simulink model "iiwa_IK_FABRIK_ROS (bkp)"  (R2016b)
settings: Solver=FixedStepAuto  StartTime=0.0  StopTime=inf  FixedStep=0.05  RelTol=1e-3
model workspace (MAT data in the model file):
  SL_ROS_VariableLengthArrays_MaxSizes.CommonInfo.ArrayTruncateAction = 'EmitWarning'
  SL_ROS_VariableLengthArrays_MaxSizes.MsgTypeMap = containers.Map
  SL_ROS_VariableLengthArrays_MaxSizes.MsgTypeMap.serialization.keys = {'nav_msgs/Path', 'sensor_msgs/JointState'}
  SL_ROS_VariableLengthArrays_MaxSizes.MsgTypeMap.serialization.values{1}.PropertyName = 'Poses'
  SL_ROS_VariableLengthArrays_MaxSizes.MsgTypeMap.serialization.values{1}.DataType = 'geometry_msgs/PoseStamped'
  SL_ROS_VariableLengthArrays_MaxSizes.MsgTypeMap.serialization.values{1}.MaxLength = 330
  SL_ROS_VariableLengthArrays_MaxSizes.MsgTypeMap.serialization.values{2}(1).PropertyName = 'Name'
  SL_ROS_VariableLengthArrays_MaxSizes.MsgTypeMap.serialization.values{2}(1).DataType = 'std_msgs/String'
  SL_ROS_VariableLengthArrays_MaxSizes.MsgTypeMap.serialization.values{2}(1).MaxLength = 30
  SL_ROS_VariableLengthArrays_MaxSizes.MsgTypeMap.serialization.values{2}(2).PropertyName = 'Position'
  SL_ROS_VariableLengthArrays_MaxSizes.MsgTypeMap.serialization.values{2}(2).DataType = 'double'
  SL_ROS_VariableLengthArrays_MaxSizes.MsgTypeMap.serialization.values{2}(2).MaxLength = 128
  SL_ROS_VariableLengthArrays_MaxSizes.MsgTypeMap.serialization.values{2}(3).PropertyName = 'Velocity'
  SL_ROS_VariableLengthArrays_MaxSizes.MsgTypeMap.serialization.values{2}(3).DataType = 'double'
  SL_ROS_VariableLengthArrays_MaxSizes.MsgTypeMap.serialization.values{2}(3).MaxLength = 128
  SL_ROS_VariableLengthArrays_MaxSizes.MsgTypeMap.serialization.values{2}(4).PropertyName = 'Effort'
  SL_ROS_VariableLengthArrays_MaxSizes.MsgTypeMap.serialization.values{2}(4).DataType = 'double'
  SL_ROS_VariableLengthArrays_MaxSizes.MsgTypeMap.serialization.values{2}(4).MaxLength = 128
  SL_ROS_VariableLengthArrays_MaxSizes.MsgTypeMap.serialization.uniformity = 0
  SL_ROS_VariableLengthArrays_MaxSizes.MsgTypeMap.serialization.keyType = 'char'
  SL_ROS_VariableLengthArrays_MaxSizes.MsgTypeMap.serialization.valueType = 'any'
libraries: robotlib x7
(part 1 of 2)
settings Model: Creator=ram  LastModifiedBy=ram

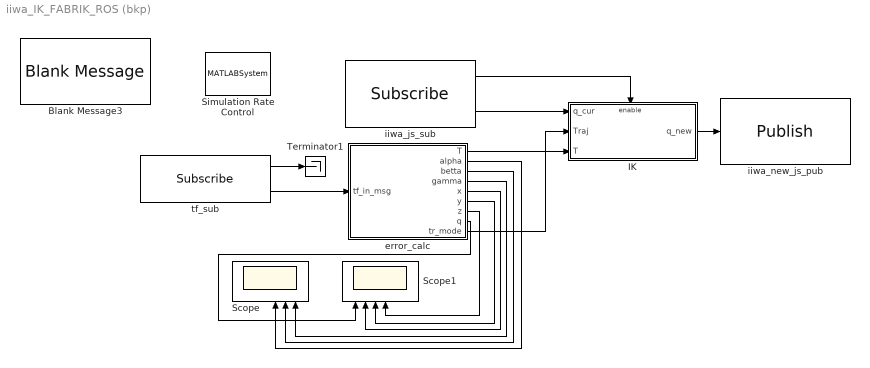
== system iiwa_IK_FABRIK_ROS (bkp) ==
  Blank Message3 : robotlib/Blank Message  SourceLibraryInfo=This block requires Robotics System Toolbox  messageType=tf2_msgs/TFMessage  SampleTime=inf
  IK : Subsystem
  Scope : Scope  NumInputPorts=6
  Scope1 : Scope  NumInputPorts=6
  Simulation Rate Control : MATLABSystem  System=ExampleHelperSimulationRateControl  SampleTime=0.05
      mask Type: ExampleHelperSimulationRateControl
      mask Display: disp('Rate Control');
  Terminator1 : Terminator
  error_calc : MATLAB Function  TreatAsAtomicUnit=on
  iiwa_js_sub : robotlib/Subscribe  SourceLibraryInfo=This block requires Robotics System Toolbox  topicSource=Select from ROS network  topic=/joint_states  messageType=sensor_msgs/JointState  sampleTime=-1  messageQueueLength=1
  iiwa_new_js_pub : robotlib/Publish  SourceLibraryInfo=This block requires Robotics System Toolbox  topicSource=Select from ROS network  topic=/arm_state  messageType=sensor_msgs/JointState  messageQueueLength=5
  tf_sub : robotlib/Subscribe  SourceLibraryInfo=This block requires Robotics System Toolbox  topicSource=Select from ROS network  topic=/tf  messageType=tf2_msgs/TFMessage  sampleTime=-1  messageQueueLength=1
  wires:
  tf_sub/2 -> error_calc/1(tf_in_msg)
  tf_sub/1 -> Terminator1/1
  iiwa_js_sub/1 -> IK/Enable
  error_calc/1(T) -> IK/3(T)
  iiwa_js_sub/2 -> IK/1(q_cur)
  IK/1(q_new) -> iiwa_new_js_pub/1
  error_calc/5(x) -> Scope1/2
  error_calc/6(y) -> Scope1/3
  error_calc/7(z) -> Scope1/4
  error_calc/2(alpha) -> Scope/4
  error_calc/3(betta) -> Scope/5
  error_calc/4(gamma) -> Scope/6
  error_calc/8(q) -> Scope1/1
  error_calc/9(tr_mode) -> IK/2(Traj)

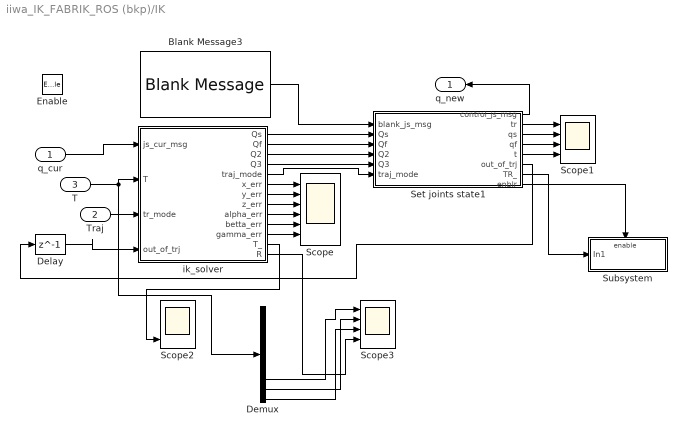
== system iiwa_IK_FABRIK_ROS (bkp)/IK ==
  q_cur : Inport
  Traj : Inport  Port=2
  T : Inport  Port=3
  Enable : EnablePort
  Blank Message3 : robotlib/Blank Message  SourceLibraryInfo=This block requires Robotics System Toolbox  messageType=sensor_msgs/JointState  SampleTime=inf
  Delay : Delay  DelayLength=1
  Demux : Demux  Outputs=10
  Scope : Scope  NumInputPorts=6
  Scope1 : Scope  NumInputPorts=4
  Scope2 : Scope  NumInputPorts=4
  Scope3 : Scope  NumInputPorts=4
  Set joints state1 : MATLAB Function  TreatAsAtomicUnit=on
  Subsystem : Subsystem
  ik_solver : MATLAB Function  TreatAsAtomicUnit=on
  q_new : Outport
  wires:
  T/1 -> Demux/1, ik_solver/2(T)
  q_cur/1 -> ik_solver/1(js_cur_msg)
  Blank Message3/1 -> Set joints state1/1(blank_js_msg)
  Set joints state1/1(control_js_msg) -> q_new/1
  ik_solver/2(Qf) -> Set joints state1/3(Qf)
  ik_solver/6(x_err) -> Scope/1
  ik_solver/7(y_err) -> Scope/2
  ik_solver/8(z_err) -> Scope/3
  ik_solver/9(alpha_err) -> Scope/4
  ik_solver/10(betta_err) -> Scope/5
  ik_solver/11(gamma_err) -> Scope/6
  Traj/1 -> ik_solver/3(tr_mode)
  ik_solver/5(traj_mode) -> Set joints state1/6(traj_mode)
  Set joints state1/6(out_of_trj) -> Delay/1
  ik_solver/1(Qs) -> Set joints state1/2(Qs)
  ik_solver/3(Q2) -> Set joints state1/4(Q2)
  ik_solver/4(Q3) -> Set joints state1/5(Q3)
  Delay/1 -> ik_solver/4(out_of_trj)
  Set joints state1/2(tr) -> Scope1/1
  Set joints state1/3(qs) -> Scope1/2
  Set joints state1/4(qf) -> Scope1/3
  Set joints state1/5(t) -> Scope1/4
  Set joints state1/7(TR_) -> Subsystem/1(In1)
  Set joints state1/8(enblr) -> Subsystem/Enable
  ik_solver/12(T_) -> Scope2/4
  ik_solver/13(R) -> Scope3/4
  Demux/10 -> Scope3/3
  Demux/8 -> Scope3/1
  Demux/9 -> Scope3/2

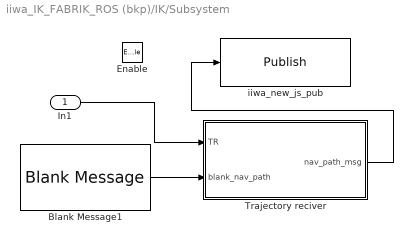
== system iiwa_IK_FABRIK_ROS (bkp)/IK/Subsystem ==
  In1 : Inport
  Enable : EnablePort
  Blank Message1 : robotlib/Blank Message  SourceLibraryInfo=This block requires Robotics System Toolbox  messageType=nav_msgs/Path  SampleTime=inf
  Trajectory reciver : MATLAB Function  TreatAsAtomicUnit=on
  iiwa_new_js_pub : robotlib/Publish  SourceLibraryInfo=This block requires Robotics System Toolbox  topicSource=Specify your own  topic=/tool_path  messageType=nav_msgs/Path  messageQueueLength=5
  wires:
  Blank Message1/1 -> Trajectory reciver/2(blank_nav_path)
  Trajectory reciver/1(nav_path_msg) -> iiwa_new_js_pub/1
  In1/1 -> Trajectory reciver/1(TR)

== matlab function iiwa_IK_FABRIK_ROS (bkp)/IK/Set joints state1 ==
  data: blank_js_msg input; Qs input; control_js_msg output Bus: SL_Bus_iiwa_IK_FABRIK_ROS_sensor_msgs_JointState; tr output; qs output; qf output; t output; Qf input double size=1 7; Q2 input; Q3 input; traj_mode input; out_of_trj output; TR_ output; enblr output
function [control_js_msg, tr, qs, qf, t, out_of_trj, TR_, enblr]   = fcn(blank_js_msg, Qs, Qf, Q2, Q3, traj_mode)

persistent on_traj;
if isempty(on_traj)
    on_traj = false;
end

persistent Qs_;
if isempty(Qs_)
    Qs_ = [0, 0, 0, 0, 0, 0];
end
qs = Qs_;
persistent Qf_;
if isempty(Qf_)
    Qf_ = [0, 0, 0, 0, 0, 0];
end
qf = Qf_;
persistent Q2_;
if isempty(Q2_)
    Q2_ = [0, 0, 0, 0, 0, 0];
end
persistent Q3_;
if isempty(Q3_)
    Q3_ = [0, 0, 0, 0, 0, 0];
end

persistent seq;
if isempty(seq)
    seq = 0;
end

persistent i;
if isempty(i)
    i = 0;
end

persistent TRth;
if isempty(TRth)
    TRth = zeros(300,6);
end

persistent TR;
if isempty(TR)
    TR = zeros(300,3);
end

enblr = 0;

out_of_trj = true;

str_array_of_jnames = {'iiwa_j1', 'iiwa_j2', 'iiwa_j3', 'iiwa_j4', 'iiwa_j5', 'iiwa_j6', 'iiwa_j7'};
control_js_msg = blank_js_msg;

th_num = length(str_array_of_jnames);
control_js_msg.Name_SL_Info.CurrentLength = uint32(th_num);

for idx=1:th_num
    str = str_array_of_jnames{idx};
    str_length = length(str);
    control_js_msg.Name(idx).Data(1:str_length) = uint8(str);
    control_js_msg.Name(idx).Data_SL_Info.CurrentLength = uint32(str_length);
end

if (traj_mode == false)
    control_js_msg.Position_SL_Info.CurrentLength = uint32(th_num);
    control_js_msg.Position(1) = double(Qf(1));
    control_js_msg.Position(2) = double(Qf(2));
    control_js_msg.Position(3) = double(Qf(3));
    control_js_msg.Position(4) = double(Qf(4));
    control_js_msg.Position(5) = double(Qf(5));
    control_js_msg.Position(6) = double(Qf(6));
    control_js_msg.Position(7) = double(Qf(7));

    control_js_msg.Header.Seq = uint32(seq);
    seq = seq + 1;
    tr = zeros(1,6);
    tr(1) = Qf(1); tr(2) = Qf(2); tr(3) = Qf(4); 
    tr(4) = Qf(5); tr(5) = Qf(6); tr(6) = Qf(7);
    t = 0;
    TR_ = zeros(300,3);
else
    if (on_traj == false)
        Qs_(1:2) = Qs(1:2); Qs_(3:6) = Qs(4:7);
        Q2_(1:2) = Q2(1:2); Q2_(3:6) = Q2(4:7);
        Q3_(1:2) = Q3(1:2); Q3_(3:6) = Q3(4:7);
        Qf_(1:2) = Qf(1:2); Qf_(3:6) = Qf(4:7);
        %%%%%%%%%%%%%%%%%%%%%%%%%%%%%%%%%%%%%%%%%%%%%%%%%%%%%
        enblr = 1;
        %TR_ = zeros(300,3);
        for j = 1:1:300
            tj = j/100;
            TRth(j,:) = traj434(2, Qs_', Q2_', Q3_', Qf_', tj);
            TR(j,:) = FK(TRth(j,1), TRth(j,2), 0.0, TRth(j,3), TRth(j,4), TRth(j,5), TRth(j,6));
            %plot3(TR(1:301,1), TR(1:301,2), TR(1:301,3));
        end
        %%%%%%%%%%%%%%%%%%%%%%%%%%%%%%%%%%%%%%%%%%%%%%%
        
        on_traj = true;
    end
    TR_ = TR;
    out_of_trj = false;
    
    t = i/100;
    tr = traj434(2, Qs_', Q2_', Q3_', Qf_', t);
    i = i + 1;
    if (i== 300)
        i = 0;
        out_of_trj = true;
        on_traj = false;
    end
    
    control_js_msg.Position_SL_Info.CurrentLength = uint32(th_num);
    control_js_msg.Position(1) = double(tr(1));
    control_js_msg.Position(2) = double(tr(2));
    control_js_msg.Position(3) = double(0.0);
    control_js_msg.Position(4) = double(tr(3));
    control_js_msg.Position(5) = double(tr(4));
    control_js_msg.Position(6) = double(tr(5));
    control_js_msg.Position(7) = double(tr(6));

    control_js_msg.Header.Seq = uint32(seq);
    seq = seq + 1;
    
end


end



function tr = traj434(in_t, in_qs, in_q2, in_q3, in_qf, t)%, in_dqs, in_dqf, in_ddqs, in_ddqf)
    
    n = 6;%numrows(in_qs);

    % Обнуление не заданных граничных условий
    %if nargin == 6 
        in_dqs  = zeros(1,n)'; in_dqf  = zeros(1,n)';
        in_ddqs = zeros(1,n)'; in_ddqf = zeros(1,n)';
    %end
    
    % интерполяция с интервалом в 10мс
    %itr_n = in_t*100;
    %t_step = 1/itr_n;
    
    % Соответствующая матрица из выражения 
    Am = [0  0  0  0  1  0  0   0   0   0   0   0   0   0;...
          0  0  0  1  0  0  0   0   0   0   0   0   0   0;...
          0  0  2  0  0  0  0   0   0   0   0   0   0   0;...
          1  1  1  1  1  0  0   0   0   0   0   0   0   0;...
          0  0  0  0  0  0  0   0   1   0   0   0   0   0;...
          4  3  2  1  0  0  0   -1  0   0   0   0   0   0;...
          12 6  2  0  0  0  -2  0   0   0   0   0   0   0;...
          0  0  0  0  0  1  1   1   1   0   0   0   0   0;...
          0  0  0  0  0  0  0   0   0   0   0   0   0   1;...
          0  0  0  0  0  3  2   1   0   0   0   0   -1  0;...
          0  0  0  0  0  6  2   0   0   0   0   -2  0   0;...
          0  0  0  0  0  0  0   0   0   1   1   1   1   1;...
          0  0  0  0  0  0  0   0   0   4   3   2   1   0;...
          0  0  0  0  0  0  0   0   0   12  6   2   0   0];
    Ami = inv(Am);
    
    % Определение полиномиальных коэффициентов для граничных условий
    % всех обобщенных координат A, скоростей dA и ускорений ddA
    A = ones(6,14);
    for i=1:n
        A(i,:)   = Ami*[in_qs(i); in_dqs(i); in_ddqs(i); in_q2(i); in_q2(i);0; 0; ...
                        in_q3(i); in_q3(i); 0; 0; in_qf(i); in_dqf(i); in_ddqf(i)];
    end
    
    % Вычисление значений интерполирующих полиномов по всей траектории
    tr = zeros(1,n);
    if t <= 1
        for i=1:n
            tr(1,i) = polyval(A(i,1:5),t);
        end
    end
    
    if (t > 1) && (t <= 2)
        for i=1:n
            tr(1,i) = polyval(A(i,6:9),(t-1));
        end
    end
    
    if (t > 2)
        for i=1:n
            tr(1,i) = polyval(A(i,10:14),(t-2));
        end
    end
end


function TRxyz = FK(th1, th2, th3, th4, th5, th6, th7)
d01 = 0.36;
d23 = 0.42;
d45 = 0.4;
d67 = 0.126;
H = [cos(th7)*(sin(th6)*(sin(th4)*(sin(th1)*sin(th3) - cos(th1)*cos(th2)*cos(th3)) - cos(th1)*cos(th4)*sin(th2)) - cos(th6)*(cos(th5)*(cos(th4)*(sin(th1)*sin(th3) - cos(th1)*cos(th2)*cos(th3)) + cos(th1)*sin(th2)*sin(th4)) + sin(th5)*(cos(th3)*sin(th1) + cos(th1)*cos(th2)*sin(th3)))) + sin(th7)*(sin(th5)*(cos(th4)*(sin(th1)*sin(th3) - cos(th1)*cos(th2)*cos(th3)) + cos(th1)*sin(th2)*sin(th4)) - cos(th5)*(cos(th3)*sin(th1) + cos(th1)*cos(th2)*sin(th3))), cos(th7)*(sin(th5)*(cos(th4)*(sin(th1)*sin(th3) - cos(th1)*cos(th2)*cos(th3)) + cos(th1)*sin(th2)*sin(th4)) - cos(th5)*(cos(th3)*sin(th1) + cos(th1)*cos(th2)*sin(th3))) - sin(th7)*(sin(th6)*(sin(th4)*(sin(th1)*sin(th3) - cos(th1)*cos(th2)*cos(th3)) - cos(th1)*cos(th4)*sin(th2)) - cos(th6)*(cos(th5)*(cos(th4)*(sin(th1)*sin(th3) - cos(th1)*cos(th2)*cos(th3)) + cos(th1)*sin(th2)*sin(th4)) + sin(th5)*(cos(th3)*sin(th1) + cos(th1)*cos(th2)*sin(th3)))),   cos(th6)*(sin(th4)*(sin(th1)*sin(th3) - cos(th1)*cos(th2)*cos(th3)) - cos(th1)*cos(th4)*sin(th2)) + sin(th6)*(cos(th5)*(cos(th4)*(sin(th1)*sin(th3) - cos(th1)*cos(th2)*cos(th3)) + cos(th1)*sin(th2)*sin(th4)) + sin(th5)*(cos(th3)*sin(th1) + cos(th1)*cos(th2)*sin(th3))),   d67*(cos(th6)*(sin(th4)*(sin(th1)*sin(th3) - cos(th1)*cos(th2)*cos(th3)) - cos(th1)*cos(th4)*sin(th2)) + sin(th6)*(cos(th5)*(cos(th4)*(sin(th1)*sin(th3) - cos(th1)*cos(th2)*cos(th3)) + cos(th1)*sin(th2)*sin(th4)) + sin(th5)*(cos(th3)*sin(th1) + cos(th1)*cos(th2)*sin(th3)))) + d45*(sin(th4)*(sin(th1)*sin(th3) - cos(th1)*cos(th2)*cos(th3)) - cos(th1)*cos(th4)*sin(th2)) - d23*cos(th1)*sin(th2);...
     -cos(th7)*(sin(th6)*(sin(th4)*(cos(th1)*sin(th3) + cos(th2)*cos(th3)*sin(th1)) + cos(th4)*sin(th1)*sin(th2)) - cos(th6)*(cos(th5)*(cos(th4)*(cos(th1)*sin(th3) + cos(th2)*cos(th3)*sin(th1)) - sin(th1)*sin(th2)*sin(th4)) + sin(th5)*(cos(th1)*cos(th3) - cos(th2)*sin(th1)*sin(th3)))) - sin(th7)*(sin(th5)*(cos(th4)*(cos(th1)*sin(th3) + cos(th2)*cos(th3)*sin(th1)) - sin(th1)*sin(th2)*sin(th4)) - cos(th5)*(cos(th1)*cos(th3) - cos(th2)*sin(th1)*sin(th3))), sin(th7)*(sin(th6)*(sin(th4)*(cos(th1)*sin(th3) + cos(th2)*cos(th3)*sin(th1)) + cos(th4)*sin(th1)*sin(th2)) - cos(th6)*(cos(th5)*(cos(th4)*(cos(th1)*sin(th3) + cos(th2)*cos(th3)*sin(th1)) - sin(th1)*sin(th2)*sin(th4)) + sin(th5)*(cos(th1)*cos(th3) - cos(th2)*sin(th1)*sin(th3)))) - cos(th7)*(sin(th5)*(cos(th4)*(cos(th1)*sin(th3) + cos(th2)*cos(th3)*sin(th1)) - sin(th1)*sin(th2)*sin(th4)) - cos(th5)*(cos(th1)*cos(th3) - cos(th2)*sin(th1)*sin(th3))), - cos(th6)*(sin(th4)*(cos(th1)*sin(th3) + cos(th2)*cos(th3)*sin(th1)) + cos(th4)*sin(th1)*sin(th2)) - sin(th6)*(cos(th5)*(cos(th4)*(cos(th1)*sin(th3) + cos(th2)*cos(th3)*sin(th1)) - sin(th1)*sin(th2)*sin(th4)) + sin(th5)*(cos(th1)*cos(th3) - cos(th2)*sin(th1)*sin(th3))), - d67*(cos(th6)*(sin(th4)*(cos(th1)*sin(th3) + cos(th2)*cos(th3)*sin(th1)) + cos(th4)*sin(th1)*sin(th2)) + sin(th6)*(cos(th5)*(cos(th4)*(cos(th1)*sin(th3) + cos(th2)*cos(th3)*sin(th1)) - sin(th1)*sin(th2)*sin(th4)) + sin(th5)*(cos(th1)*cos(th3) - cos(th2)*sin(th1)*sin(th3)))) - d45*(sin(th4)*(cos(th1)*sin(th3) + cos(th2)*cos(th3)*sin(th1)) + cos(th4)*sin(th1)*sin(th2)) - d23*sin(th1)*sin(th2);...
     cos(th7)*(cos(th6)*(cos(th5)*(cos(th2)*sin(th4) + cos(th3)*cos(th4)*sin(th2)) - sin(th2)*sin(th3)*sin(th5)) + sin(th6)*(cos(th2)*cos(th4) - cos(th3)*sin(th2)*sin(th4))) - sin(th7)*(sin(th5)*(cos(th2)*sin(th4) + cos(th3)*cos(th4)*sin(th2)) + cos(th5)*sin(th2)*sin(th3)),                                                                                                                                                                                     - cos(th7)*(sin(th5)*(cos(th2)*sin(th4) + cos(th3)*cos(th4)*sin(th2)) + cos(th5)*sin(th2)*sin(th3)) - sin(th7)*(cos(th6)*(cos(th5)*(cos(th2)*sin(th4) + cos(th3)*cos(th4)*sin(th2)) - sin(th2)*sin(th3)*sin(th5)) + sin(th6)*(cos(th2)*cos(th4) - cos(th3)*sin(th2)*sin(th4))),                                                                                                                  cos(th6)*(cos(th2)*cos(th4) - cos(th3)*sin(th2)*sin(th4)) - sin(th6)*(cos(th5)*(cos(th2)*sin(th4) + cos(th3)*cos(th4)*sin(th2)) - sin(th2)*sin(th3)*sin(th5)),                                                                                                                                                             d01 + d45*(cos(th2)*cos(th4) - cos(th3)*sin(th2)*sin(th4)) - d67*(sin(th6)*(cos(th5)*(cos(th2)*sin(th4) + cos(th3)*cos(th4)*sin(th2)) - sin(th2)*sin(th3)*sin(th5)) - cos(th6)*(cos(th2)*cos(th4) - cos(th3)*sin(th2)*sin(th4))) + d23*cos(th2);...
                                                                                                                                                                                                                                                                                                                                                                                                                                                                        0,                                                                                                                                                                                                                                                                                                                                                                                                                                                                  0,                                                                                                                                                                                                                                                                              0,                                                                                                                                                                                                                                                                                                                                                                                                           1];  
TRxyz = H*[0;0;0;1];
TRxyz = TRxyz(1:3,1)';
end



function tr = traj434all(in_t, in_qs, in_q2, in_q3, in_qf)%, in_dqs, in_dqf, in_ddqs, in_ddqf)
    
    n = 6;%numrows(in_qs);

    % Обнуление не заданных граничных условий
    %if nargin == 6 
        in_dqs  = zeros(1,n)'; in_dqf  = zeros(1,n)';
        in_ddqs = zeros(1,n)'; in_ddqf = zeros(1,n)';
    %end
    
    % интерполяция с интервалом в 10мс
    itr_n = in_t*100;
    t_step = 1/itr_n;
    
    % Соответствующая матрица из выражения 
    Am = [0  0  0  0  1  0  0   0   0   0   0   0   0   0;...
          0  0  0  1  0  0  0   0   0   0   0   0   0   0;...
          0  0  2  0  0  0  0   0   0   0   0   0   0   0;...
          1  1  1  1  1  0  0   0   0   0   0   0   0   0;...
          0  0  0  0  0  0  0   0   1   0   0   0   0   0;...
          4  3  2  1  0  0  0   -1  0   0   0   0   0   0;...
          12 6  2  0  0  0  -2  0   0   0   0   0   0   0;...
          0  0  0  0  0  1  1   1   1   0   0   0   0   0;...
          0  0  0  0  0  0  0   0   0   0   0   0   0   1;...
          0  0  0  0  0  3  2   1   0   0   0   0   -1  0;...
          0  0  0  0  0  6  2   0   0   0   0   -2  0   0;...
          0  0  0  0  0  0  0   0   0   1   1   1   1   1;...
          0  0  0  0  0  0  0   0   0   4   3   2   1   0;...
          0  0  0  0  0  0  0   0   0   12  6   2   0   0];
    Ami = inv(Am);
    
    % Определение полиномиальных коэффициентов для граничных условий
    % всех обобщенных координат A, скоростей dA и ускорений ddA
    A = ones(6,14);
    for i=1:n
        A(i,:)   = Ami*[in_qs(i); in_dqs(i); in_ddqs(i); in_q2(i); in_q2(i);0; 0; ...
                        in_q3(i); in_q3(i); 0; 0; in_qf(i); in_dqf(i); in_ddqf(i)];
        %dA(i,:)  = polyder(A(i,:));
        %ddA(i,:) = polyder(dA(i,:));
    end
    nt = (0:t_step:1);
    nn = size(nt);

    tr = zeros(nn(2),n);

    % Вычисление значений интерполирующих полиномов по всей траектории
    for i=1:n
        itr = 1;
        for t=0:t_step:1
            tr(itr, i, 1) = polyval(A(i,:),t);
            itr = itr + 1;
        end
    end
end

== matlab function iiwa_IK_FABRIK_ROS (bkp)/IK/Subsystem/Trajectory reciver ==
  data: TR input; blank_nav_path input; nav_path_msg output Bus: SL_Bus_iiwa_IK_FABRIK_ROS_nav_msgs_Path
function nav_path_msg = fcn(TR, blank_nav_path)

persistent seq;
if isempty(seq)
    seq = 0;
end


par_frame = 'iiwa_base_link';
par_fr_n = length(par_frame);

nav_path_msg = blank_nav_path;
nav_path_msg.Header.Seq = uint32(seq);
nav_path_msg.Header.FrameId_SL_Info.CurrentLength = uint32(par_fr_n);
nav_path_msg.Header.FrameId(1:par_fr_n) = uint8(par_frame);

s = size(TR);

p_num = s(1,1);
nav_path_msg.Poses_SL_Info.CurrentLength = uint32(p_num);

for idx=1:p_num
    x = TR(idx,1);
    y = TR(idx,2);
    z = TR(idx,3);
    nav_path_msg.Poses(idx).Header.Seq = uint32(seq*300 + idx);
    nav_path_msg.Poses(idx).Header.FrameId_SL_Info.CurrentLength = uint32(par_fr_n);
    nav_path_msg.Poses(idx).Header.FrameId(1:par_fr_n) = uint8(par_frame);
    nav_path_msg.Poses(idx).Pose.Position.X = double(x);
    nav_path_msg.Poses(idx).Pose.Position.Y = double(y);
    nav_path_msg.Poses(idx).Pose.Position.Z = double(z);
    nav_path_msg.Poses(idx).Pose.Orientation.X = double(0.0);
    nav_path_msg.Poses(idx).Pose.Orientation.Y = double(0.0);
    nav_path_msg.Poses(idx).Pose.Orientation.Z = double(0.0);
    nav_path_msg.Poses(idx).Pose.Orientation.W = double(1.0);
end

seq = seq + 1;


end
